simulink model "msd_02_Simulink_2"  (R2014a)
settings: Solver=ode45  StartTime=0.0  StopTime=10.0  RelTol=1e-3
undefined symbols (not defined in the file): b, k, m
Description:
  | Copyright 2014 The MathWorks, Inc.
settings Model: Creator=smiller  LastModifiedBy=smiller
settings DebuggingCC: UnderspecifiedInitializationDetection=Classic  StateNameClashWarn=warning

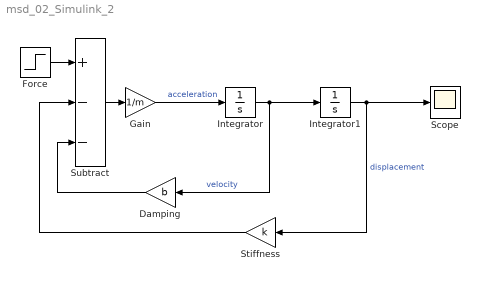
== system msd_02_Simulink_2 ==
  Damping : Gain  Gain=b
  Force : Step  After=10  SampleTime=0
  Gain : Gain  Gain=1/m
  Integrator : Integrator
  Integrator1 : Integrator
  Scope : Scope
  Stiffness : Gain  Gain=k
  Subtract : Sum  Inputs=+--
  wires:
  Force/1 -> Subtract/1
  Subtract/1 -> Gain/1
  Gain/1 -> Integrator/1  "acceleration"
  Integrator/1 -> Damping/1, Integrator1/1  "velocity"
  Stiffness/1 -> Subtract/2
  Damping/1 -> Subtract/3
  Integrator1/1 -> Scope/1, Stiffness/1  "displacement"
